simulink model "Es2"  (R2021a)
settings: Solver=VariableStepAuto  StartTime=0.0  StopTime=60  RelTol=1e-3
undefined symbols (not defined in the file or in its folder): gravload, Kd, Kp, p560_nofric, qql, qqr
settings Model: Creator=Andrea  LastModifiedBy=mular
settings SolverCC: AlgebraicLoopSolver=TrustRegion
settings DataIOCC: ReturnWorkspaceOutputs=off
settings DebuggingCC: SFMachineParentedDataDiag=warning  ArithmeticOperatorsInVariantConditions=warning
settings SFSimCC: CustomCodeUndefinedFunction=UseInterfaceOnly

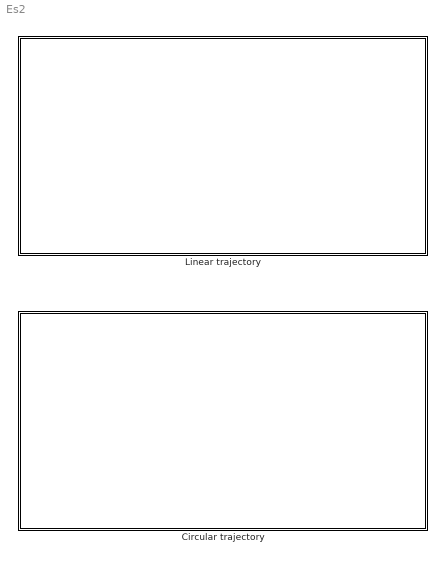
== system Es2 ==
  Circular trajectory : Subsystem
  Linear trajectory : Subsystem

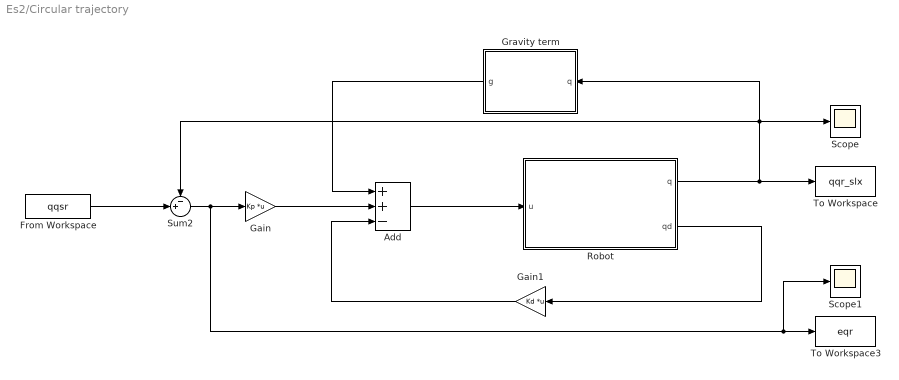
== system Es2/Circular trajectory ==
  Add : Sum  Inputs=++-
  From Workspace : FromWorkspace  VariableName=qqsr  OutputAfterFinalValue=Holding final value
  Gain : Gain  Gain=Kp  Multiplication=Matrix(K*u)
  Gain1 : Gain  Gain=Kd  Multiplication=Matrix(K*u)
  Gravity term : Subsystem  mask{robot=p560_nofric}
  Robot : Subsystem  mask{robot=p560_nofric, q0=qqr(1,:)}
      mask prompts: robot "Robot object"; q0 "Initial state"
  Scope : Scope
  Scope1 : Scope
  Sum2 : Sum  Inputs=-+|
  To Workspace : ToWorkspace  VariableName=qqr_slx  SaveFormat=Timeseries  SampleTime=-1
  To Workspace3 : ToWorkspace  VariableName=eqr  SaveFormat=Timeseries  SampleTime=-1
  wires:
  Gravity term/1(g) -> Add/1
  Gain/1 -> Add/2
  Add/1 -> Robot/1(u)
  Gain1/1 -> Add/3
  Sum2/1 -> Gain/1, Scope1/1, To Workspace3/1
  Robot/1(q) -> Sum2/1, Gravity term/1(q), Scope/1, To Workspace/1
  Robot/2(qd) -> Gain1/1
  From Workspace/1 -> Sum2/2

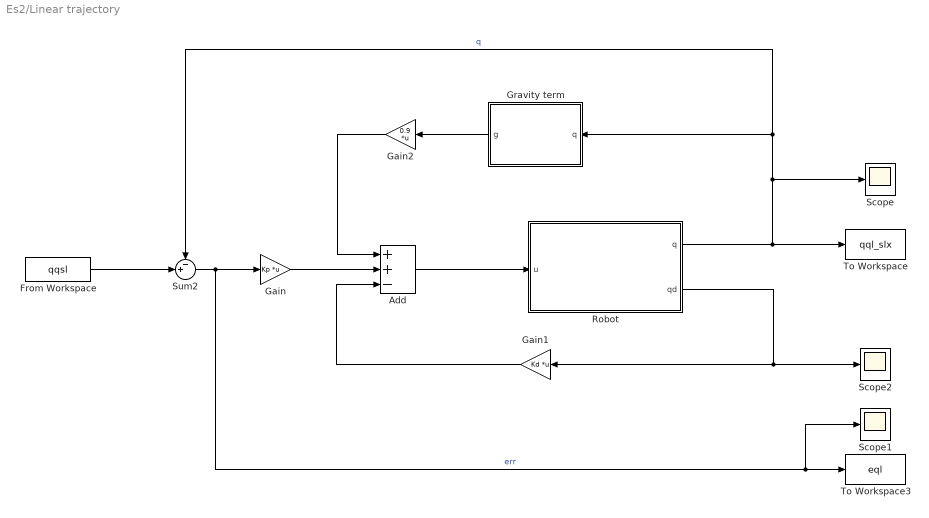
== system Es2/Linear trajectory ==
  Add : Sum  Inputs=++-
  From Workspace : FromWorkspace  VariableName=qqsl  OutputAfterFinalValue=Holding final value
  Gain : Gain  Gain=Kp  Multiplication=Matrix(K*u)
  Gain1 : Gain  Gain=Kd  Multiplication=Matrix(K*u)
  Gain2 : Gain  Gain=0.9  Multiplication=Matrix(K*u)
  Gravity term : Subsystem  mask{robot=p560_nofric}
  Robot : Subsystem  mask{robot=p560_nofric, q0=qql(1,:)}
      mask prompts: robot "Robot object"; q0 "Initial state"
  Scope : Scope
  Scope1 : Scope
  Scope2 : Scope
  Sum2 : Sum  Inputs=-+|
  To Workspace : ToWorkspace  VariableName=qql_slx  SaveFormat=Timeseries  SampleTime=-1
  To Workspace3 : ToWorkspace  VariableName=eql  SaveFormat=Timeseries  SampleTime=-1
  wires:
  Sum2/1 -> Scope1/1, To Workspace3/1, Gain/1  "err"
  Gain1/1 -> Add/3
  Add/1 -> Robot/1(u)
  Gain/1 -> Add/2
  Gravity term/1(g) -> Gain2/1
  Robot/2(qd) -> Gain1/1, Scope2/1
  Robot/1(q) -> Sum2/1, Gravity term/1(q), Scope/1, To Workspace/1  "q"
  From Workspace/1 -> Sum2/2
  Gain2/1 -> Add/1

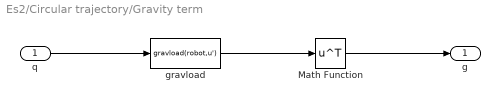
== system Es2/Circular trajectory/Gravity term ==
  q : Inport
  Math Function : Math  Operator=transpose  SignedPower=on  SaturateOnIntegerOverflow=on
  gravload : MATLABFcn  MATLABFcn=gravload(robot,u')  OutputDimensions=[1 robot.n]  Output1D=off
  g : Outport  VectorParamsAs1DForOutWhenUnconnected=off
  wires:
  Math Function/1 -> g/1
  gravload/1 -> Math Function/1
  q/1 -> gravload/1

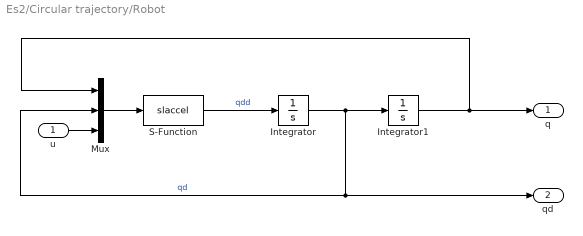
== system Es2/Circular trajectory/Robot ==
  u : Inport
  Integrator : Integrator
  Integrator1 : Integrator  InitialCondition=q0
  Mux : Mux  Inputs=3
  S-Function : S-Function  FunctionName=slaccel  Parameters=p560_nofric  SFunctionDeploymentMode=off  EnableBusSupport=off
  q : Outport  VectorParamsAs1DForOutWhenUnconnected=off
  qd : Outport  Port=2  VectorParamsAs1DForOutWhenUnconnected=off
  wires:
  u/1 -> Mux/3
  Integrator/1 -> Integrator1/1, Mux/2, qd/1  "qd"
  Mux/1 -> S-Function/1
  Integrator1/1 -> Mux/1, q/1
  S-Function/1 -> Integrator/1  "qdd"

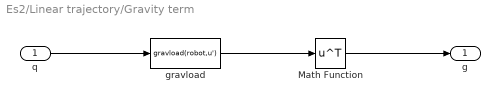
== system Es2/Linear trajectory/Gravity term ==
  q : Inport
  Math Function : Math  Operator=transpose  SignedPower=on  SaturateOnIntegerOverflow=on
  gravload : MATLABFcn  MATLABFcn=gravload(robot,u')  OutputDimensions=[1 robot.n]  Output1D=off
  g : Outport  VectorParamsAs1DForOutWhenUnconnected=off
  wires:
  q/1 -> gravload/1
  gravload/1 -> Math Function/1
  Math Function/1 -> g/1

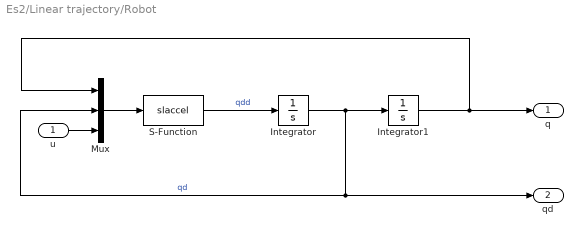
== system Es2/Linear trajectory/Robot ==
  u : Inport
  Integrator : Integrator
  Integrator1 : Integrator  InitialCondition=q0
  Mux : Mux  Inputs=3
  S-Function : S-Function  FunctionName=slaccel  Parameters=p560_nofric  SFunctionDeploymentMode=off  EnableBusSupport=off
  q : Outport  VectorParamsAs1DForOutWhenUnconnected=off
  qd : Outport  Port=2  VectorParamsAs1DForOutWhenUnconnected=off
  wires:
  S-Function/1 -> Integrator/1  "qdd"
  Integrator1/1 -> q/1, Mux/1
  Mux/1 -> S-Function/1
  Integrator/1 -> qd/1, Mux/2, Integrator1/1  "qd"
  u/1 -> Mux/3
